simulink model "slrt_pmsm_2level_inverter"  (R2022b)
settings: Solver=FixedStepAuto  StartTime=0.0  StopTime=0.25  RelTol=1e-3  EnableMultiTasking=on
PreLoadFcn:
  | Ts = 1e-4;
  | Tcpu = 50e-6; %Controller sample time
  | 
  | % PMSM parameters
  | PM = 0.03; % Permanent magnet flux linkage
  | Ld = 2e-4;  % d-axis inductance
  | Lq = 2e-4;  % q-axis inductance
  | L0 = 2e-4;  % 0-axis inductance
  | Rs = 0.013; % Stator resistance
  | N = 6; % Number of pole pairs
  | J = 0.2; % Moment of inertia
  | 
  | % encoder parameters
  | numSlits = 2000; % number of slits
  | pulseSigOffset = 0; % index pulse signal offset
  | shaftInitPos = 0; % motor shaft initial position
  | 
  | % DAC parameters
  | gain = 0.1;
  | bias = 0;
  | 
  | % circuit parameters
  | Vdc = 48;
  | 
  | % real-time parameters
  | ts_FPGA_clk = 5e-9;
  | ts_FPGA_mdl = 1e-6;
  | 
  | % Real-time processor or embedded controller
  | RTorTTL = 1; % 1: Real-time processor,    0: embedded controller
  | 
  | % sample times
  | f_base = 200e6;
  | PWM_frequency = 20e3;
  | ts_FPGA_clk = 1/f_base;
  | ts_FPGA_mdl =1e-6;
libraries: simulink x5, hdlsllib x3, mcbhdlplantlib x2, slrtencoderlib x2, slrtresolverlib x2, slrthdlutillib x1, slrt2levelinverterlib x1
settings Model: Creator=chrisz  LastModifiedBy=chrisz
settings OptimizationCC: BlockReduction=off  ConditionallyExecuteInputs=off  DefaultParameterBehavior=Inlined
settings DebuggingCC: AlgebraicLoopMsg=error  SingleTaskRateTransMsg=error
settings HardwareCC: ProdBitPerPointer=32  ProdBitPerSizeT=32  ProdBitPerPtrDiffT=32  ProdLargestAtomicFloat=None  ProdIntDivRoundTo=Undefined  ProdEndianess=Unspecified  ProdWordSize=32  ProdHWDeviceType=ASIC/FPGA->ASIC/FPGA  TargetBitPerPointer=64  TargetBitPerSizeT=64  TargetBitPerPtrDiffT=64  TargetLongLongMode=on  TargetIntDivRoundTo=Zero  TargetEndianess=LittleEndian  TargetWordSize=64  TargetHWDeviceType=Custom Processor->MATLAB Host Computer  ProdEqTarget=off
settings ModelReferenceCC: EnableRefExpFcnMdlSchedulingChecks=on

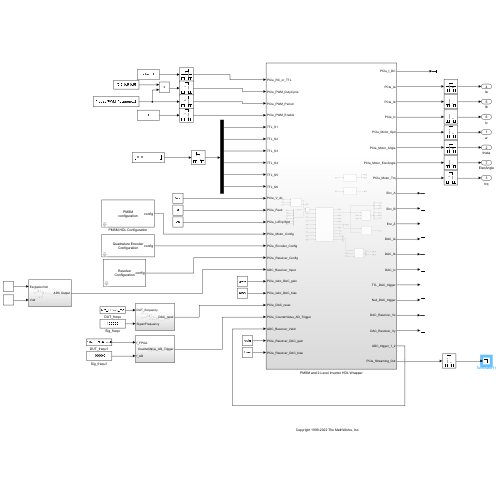
[thumbnail: Simulink's stored preview of the top-level diagram]
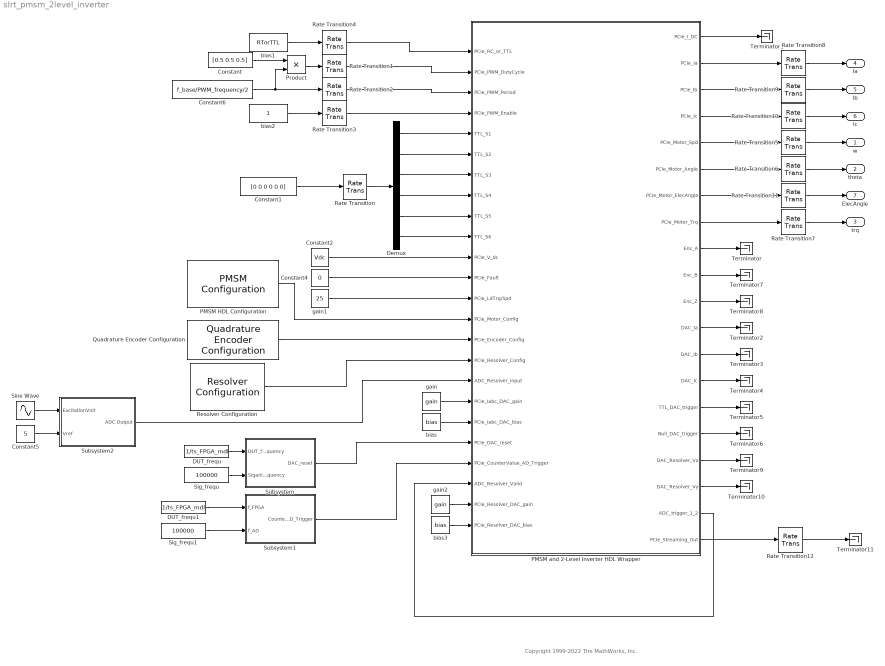
== system slrt_pmsm_2level_inverter ==
  note: Copyright 1999-2022 The MathWorks, Inc.
  Constant : Constant  Value=[0.5 0.5 0.5]  OutDataTypeStr=single  SampleTime=ts_FPGA_mdl
  Constant1 : Constant  Value=[0 0 0 0 0 0]  OutDataTypeStr=boolean  SampleTime=-1
  Constant2 : Constant  Value=Vdc  OutDataTypeStr=single  SampleTime=ts_FPGA_mdl
  Constant4 : Constant  Value=0  OutDataTypeStr=uint32  SampleTime=ts_FPGA_mdl
  Constant5 : Constant  Value=5  SampleTime=ts_FPGA_mdl
  Constant6 : Constant  Value=f_base/PWM_frequency/2  OutDataTypeStr=uint32  SampleTime=ts_FPGA_mdl
  DUT_frequ : Constant  Value=1/ts_FPGA_mdl  SampleTime=ts_FPGA_mdl
  DUT_frequ1 : Constant  Value=1/ts_FPGA_mdl  SampleTime=ts_FPGA_mdl
  Demux : Demux  Outputs=6
  PMSM HDL Configuration : mcbhdlplantlib/PMSM Configuration  portConfig=Torque  Trq_N_mode=0  Ts=1e-6  Pp=6  Rs=0.013  Ld=2e-4  Lq=2e-4  lambda_pm=0.03  J=0.2  B=4.924e-4  f=0
  PMSM and 2-Level Inverter HDL Wrapper : Subsystem
  Product : Product  OutDataTypeStr=uint32
  Quadrature Encoder Configuration : slrtencoderlib/Quadrature Encoder Configuration  NPulses=2000  zOffset=0  Ts=1e-6
  Rate Transition{,1..4} (5 alike) : RateTransition  OutPortSampleTime=ts_FPGA_clk
  Rate Transition{5..12} (8 alike) : RateTransition  OutPortSampleTime=Tcpu
  Resolver Configuration : slrtresolverlib/Resolver Configuration  Ts=1e-6  R=0.5  N=1  ADCrefV=5  ADCbits=16  totalADCCounts=65536
  Sig_frequ : Constant  Value=100000  VectorParams1D=off  SampleTime=ts_FPGA_mdl
  Sig_frequ1 : Constant  Value=100000  VectorParams1D=off  SampleTime=ts_FPGA_mdl
  Sine Wave : Sin  Amplitude=5  Frequency=62830  SampleTime=ts_FPGA_mdl
  Subsystem : Subsystem
  Subsystem1 : Subsystem
  Subsystem2 : Subsystem
  Terminator{,1..11} (12 alike) : Terminator
  bias : Constant  Value=bias  OutDataTypeStr=single  SampleTime=ts_FPGA_mdl
  bias1 : Constant  Value=RTorTTL  OutDataTypeStr=single  SampleTime=ts_FPGA_mdl
  bias2 : Constant  OutDataTypeStr=boolean  SampleTime=ts_FPGA_mdl
  bias3 : Constant  Value=bias  OutDataTypeStr=single  SampleTime=ts_FPGA_mdl
  gain : Constant  Value=gain  OutDataTypeStr=single  SampleTime=ts_FPGA_mdl
  gain1 : Constant  Value=25  OutDataTypeStr=single  SampleTime=ts_FPGA_mdl
  gain2 : Constant  Value=gain  OutDataTypeStr=single  SampleTime=ts_FPGA_mdl
  w : Outport
  theta : Outport  Port=2
  trq : Outport  Port=3
  Ia : Outport  Port=4
  Ib : Outport  Port=5
  Ic : Outport  Port=6
  ElecAngle : Outport  Port=7
  wires:
  bias1/1 -> Rate Transition4/1
  bias2/1 -> Rate Transition3/1
  Constant6/1 -> Product/2, Rate Transition2/1
  Product/1 -> Rate Transition1/1
  Constant/1 -> Product/1
  gain/1 -> PMSM and 2-Level Inverter HDL Wrapper/18(PCIe_Iabc_DAC_gain)
  bias/1 -> PMSM and 2-Level Inverter HDL Wrapper/19(PCIe_Iabc_DAC_bias)
  Rate Transition4/1 -> PMSM and 2-Level Inverter HDL Wrapper/1(PCIe_RC_or_TTL)
  Rate Transition3/1 -> PMSM and 2-Level Inverter HDL Wrapper/4(PCIe_PWM_Enable)
  Rate Transition2/1 -> PMSM and 2-Level Inverter HDL Wrapper/3(PCIe_PWM_Period)
  Rate Transition1/1 -> PMSM and 2-Level Inverter HDL Wrapper/2(PCIe_PWM_DutyCycle)
  Rate Transition/1 -> Demux/1
  Demux/1 -> PMSM and 2-Level Inverter HDL Wrapper/5(TTL_S1)
  Demux/2 -> PMSM and 2-Level Inverter HDL Wrapper/6(TTL_S2)
  Demux/3 -> PMSM and 2-Level Inverter HDL Wrapper/7(TTL_S3)
  Demux/4 -> PMSM and 2-Level Inverter HDL Wrapper/8(TTL_S4)
  Demux/5 -> PMSM and 2-Level Inverter HDL Wrapper/9(TTL_S5)
  Demux/6 -> PMSM and 2-Level Inverter HDL Wrapper/10(TTL_S6)
  Constant1/1 -> Rate Transition/1
  Constant2/1 -> PMSM and 2-Level Inverter HDL Wrapper/11(PCIe_V_dc)
  Constant4/1 -> PMSM and 2-Level Inverter HDL Wrapper/12(PCIe_Fault)
  gain1/1 -> PMSM and 2-Level Inverter HDL Wrapper/13(PCIe_LdTrq/Spd)
  DUT_frequ/1 -> Subsystem/1(DUT_frequency)
  Sig_frequ/1 -> Subsystem/2(SiganlFrequency)
  Subsystem/1(DAC_reset) -> PMSM and 2-Level Inverter HDL Wrapper/20(PCIe_DAC_reset)
  Rate Transition6/1 -> theta/1
  PMSM and 2-Level Inverter HDL Wrapper/9(Enc_A) -> Terminator/1
  Rate Transition7/1 -> trq/1
  PMSM and 2-Level Inverter HDL Wrapper/12(DAC_Ia) -> Terminator2/1
  PMSM and 2-Level Inverter HDL Wrapper/1(PCIe_I_DC) -> Terminator1/1
  PMSM and 2-Level Inverter HDL Wrapper/10(Enc_B) -> Terminator7/1
  PMSM and 2-Level Inverter HDL Wrapper/14(DAC_Ic) -> Terminator4/1
  Rate Transition5/1 -> w/1
  Rate Transition10/1 -> Ic/1
  PMSM and 2-Level Inverter HDL Wrapper/15(TTL_DAC_trigger) -> Terminator5/1
  PMSM and 2-Level Inverter HDL Wrapper/13(DAC_Ib) -> Terminator3/1
  PMSM and 2-Level Inverter HDL Wrapper/16(Null_DAC_trigger) -> Terminator6/1
  Rate Transition9/1 -> Ib/1
  Rate Transition8/1 -> Ia/1
  PMSM and 2-Level Inverter HDL Wrapper/5(PCIe_Motor_Spd) -> Rate Transition5/1
  PMSM and 2-Level Inverter HDL Wrapper/6(PCIe_Motor_Angle) -> Rate Transition6/1
  PMSM and 2-Level Inverter HDL Wrapper/8(PCIe_Motor_Trq) -> Rate Transition7/1
  PMSM and 2-Level Inverter HDL Wrapper/2(PCIe_Ia) -> Rate Transition8/1
  PMSM and 2-Level Inverter HDL Wrapper/3(PCIe_Ib) -> Rate Transition9/1
  PMSM and 2-Level Inverter HDL Wrapper/4(PCIe_Ic) -> Rate Transition10/1
  PMSM and 2-Level Inverter HDL Wrapper/11(Enc_Z) -> Terminator8/1
  PMSM and 2-Level Inverter HDL Wrapper/17(DAC_Resolver_Vx) -> Terminator9/1
  PMSM and 2-Level Inverter HDL Wrapper/18(DAC_Resolver_Vy) -> Terminator10/1
  Quadrature Encoder Configuration/1 -> PMSM and 2-Level Inverter HDL Wrapper/15(PCIe_Encoder_Config)
  PMSM HDL Configuration/1 -> PMSM and 2-Level Inverter HDL Wrapper/14(PCIe_Motor_Config)
  Resolver Configuration/1 -> PMSM and 2-Level Inverter HDL Wrapper/16(PCIe_Resolver_Config)
  Subsystem1/1(CounterValue_AD_Trigger) -> PMSM and 2-Level Inverter HDL Wrapper/21(PCIe_CounterValue_AD_Trigger)
  PMSM and 2-Level Inverter HDL Wrapper/19(ADC_trigger_1_2) -> PMSM and 2-Level Inverter HDL Wrapper/22(ADC_Resolver_Valid)
  Sig_frequ1/1 -> Subsystem1/2(f_AD)
  DUT_frequ1/1 -> Subsystem1/1(f_FPGA)
  Sine Wave/1 -> Subsystem2/1(ExcitationVolt)
  Constant5/1 -> Subsystem2/2(Vref)
  Subsystem2/1(ADC Output) -> PMSM and 2-Level Inverter HDL Wrapper/17(ADC_Resolver_Input)
  Rate Transition11/1 -> ElecAngle/1
  PMSM and 2-Level Inverter HDL Wrapper/7(PCIe_Motor_ElecAngle) -> Rate Transition11/1
  gain2/1 -> PMSM and 2-Level Inverter HDL Wrapper/23(PCIe_Resolver_DAC_gain)
  bias3/1 -> PMSM and 2-Level Inverter HDL Wrapper/24(PCIe_Resolver_DAC_bias)
  PMSM and 2-Level Inverter HDL Wrapper/20(PCIe_Streaming_Out) -> Rate Transition12/1
  Rate Transition12/1 -> Terminator11/1

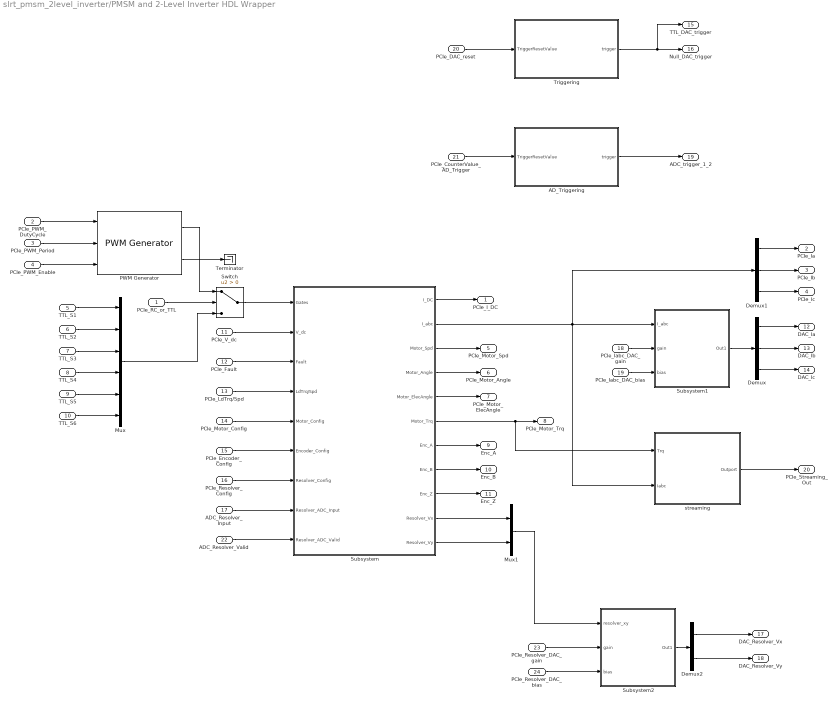
== system slrt_pmsm_2level_inverter/PMSM and 2-Level Inverter HDL Wrapper ==
  PCIe_RC_or_TTL : Inport
  PCIe_PWM_DutyCycle : Inport  Port=2
  PCIe_PWM_Period : Inport  Port=3
  PCIe_PWM_Enable : Inport  Port=4
  TTL_S1 : Inport  Port=5
  TTL_S2 : Inport  Port=6
  TTL_S3 : Inport  Port=7
  TTL_S4 : Inport  Port=8
  TTL_S5 : Inport  Port=9
  TTL_S6 : Inport  Port=10
  PCIe_V_dc : Inport  Port=11
  PCIe_Fault : Inport  Port=12
  PCIe_LdTrq/Spd : Inport  Port=13
  PCIe_Motor_Config : Inport  Port=14
  PCIe_Encoder_Config : Inport  Port=15
  PCIe_Resolver_Config : Inport  Port=16
  ADC_Resolver_Input : Inport  Port=17
  PCIe_Iabc_DAC_gain : Inport  Port=18
  PCIe_Iabc_DAC_bias : Inport  Port=19
  PCIe_DAC_reset : Inport  Port=20
  PCIe_CounterValue_AD_Trigger : Inport  Port=21  OutDataTypeStr=uint32
  ADC_Resolver_Valid : Inport  Port=22
  PCIe_Resolver_DAC_gain : Inport  Port=23
  PCIe_Resolver_DAC_bias : Inport  Port=24
  AD_Triggering : Subsystem
  Demux : Demux  Outputs=3
  Demux1 : Demux  Outputs=3
  Demux2 : Demux  Outputs=2
  Mux : Mux  Inputs=6
  Mux1 : Mux  Inputs=2
  PWM Generator : slrthdlutillib/PWM Generator
  Subsystem : Subsystem
  Subsystem1 : Subsystem
  Subsystem2 : Subsystem
  Switch : Switch  Criteria=u2 > Threshold  SaturateOnIntegerOverflow=off  InputSameDT=off
  Terminator : Terminator
  Triggering : Subsystem
  streaming : Subsystem
  PCIe_I_DC : Outport
  PCIe_Ia : Outport  Port=2
  PCIe_Ib : Outport  Port=3
  PCIe_Ic : Outport  Port=4
  PCIe_Motor_Spd : Outport  Port=5
  PCIe_Motor_Angle : Outport  Port=6
  PCIe_Motor_ElecAngle : Outport  Port=7
  PCIe_Motor_Trq : Outport  Port=8
  Enc_A : Outport  Port=9
  Enc_B : Outport  Port=10
  Enc_Z : Outport  Port=11
  DAC_Ia : Outport  Port=12
  DAC_Ib : Outport  Port=13
  DAC_Ic : Outport  Port=14
  TTL_DAC_trigger : Outport  Port=15
  Null_DAC_trigger : Outport  Port=16
  DAC_Resolver_Vx : Outport  Port=17
  DAC_Resolver_Vy : Outport  Port=18
  ADC_trigger_1_2 : Outport  Port=19  OutDataTypeStr=boolean
  PCIe_Streaming_Out : Outport  Port=20
  wires:
  Subsystem/7(Enc_A) -> Enc_A/1
  TTL_S2/1 -> Mux/2
  Demux1/1 -> PCIe_Ia/1
  PCIe_PWM_DutyCycle/1 -> PWM Generator/1
  TTL_S5/1 -> Mux/5
  Subsystem/2(I_abc) -> Demux1/1, streaming/2(Iabc), Subsystem1/1(I_abc)
  Subsystem/6(Motor_Trq) -> streaming/1(Trq), PCIe_Motor_Trq/1
  Subsystem/4(Motor_Angle) -> PCIe_Motor_Angle/1
  Subsystem/1(I_DC) -> PCIe_I_DC/1
  PCIe_Encoder_Config/1 -> Subsystem/6(Encoder_Config)
  PCIe_Iabc_DAC_bias/1 -> Subsystem1/3(bias)
  Subsystem/3(Motor_Spd) -> PCIe_Motor_Spd/1
  Subsystem/8(Enc_B) -> Enc_B/1
  PCIe_V_dc/1 -> Subsystem/2(V_dc)
  PWM Generator/1 -> Switch/1
  Triggering/1(trigger) -> Null_DAC_trigger/1, TTL_DAC_trigger/1
  TTL_S6/1 -> Mux/6
  Subsystem/9(Enc_Z) -> Enc_Z/1
  PCIe_LdTrq/Spd/1 -> Subsystem/4(LdTrq/Spd)
  TTL_S1/1 -> Mux/1
  Demux1/3 -> PCIe_Ic/1
  Demux1/2 -> PCIe_Ib/1
  PCIe_RC_or_TTL/1 -> Switch/2
  PCIe_Motor_Config/1 -> Subsystem/5(Motor_Config)
  Demux/1 -> DAC_Ia/1
  Mux/1 -> Switch/3
  PCIe_PWM_Period/1 -> PWM Generator/2
  TTL_S4/1 -> Mux/4
  PCIe_Fault/1 -> Subsystem/3(Fault)
  PCIe_DAC_reset/1 -> Triggering/1(TriggerResetValue)
  PCIe_Iabc_DAC_gain/1 -> Subsystem1/2(gain)
  PCIe_PWM_Enable/1 -> PWM Generator/3
  Demux/2 -> DAC_Ib/1
  Switch/1 -> Subsystem/1(Gates)
  Subsystem1/1(Out1) -> Demux/1
  TTL_S3/1 -> Mux/3
  Demux/3 -> DAC_Ic/1
  PCIe_Resolver_Config/1 -> Subsystem/7(Resolver_Config)
  ADC_Resolver_Input/1 -> Subsystem/8(Resolver_ADC_Input)
  PCIe_CounterValue_AD_Trigger/1 -> AD_Triggering/1(TriggerResetValue)
  AD_Triggering/1(trigger) -> ADC_trigger_1_2/1
  ADC_Resolver_Valid/1 -> Subsystem/9(Resolver_ADC_Valid)
  Subsystem/5(Motor_ElecAngle) -> PCIe_Motor_ElecAngle/1
  streaming/1(Outport) -> PCIe_Streaming_Out/1
  Subsystem/10(Resolver_Vx) -> Mux1/1
  Subsystem/11(Resolver_Vy) -> Mux1/2
  Mux1/1 -> Subsystem2/1(resolver_xy)
  PCIe_Resolver_DAC_gain/1 -> Subsystem2/2(gain)
  PCIe_Resolver_DAC_bias/1 -> Subsystem2/3(bias)
  Subsystem2/1(Out1) -> Demux2/1
  Demux2/1 -> DAC_Resolver_Vx/1
  Demux2/2 -> DAC_Resolver_Vy/1
  PWM Generator/2 -> Terminator/1

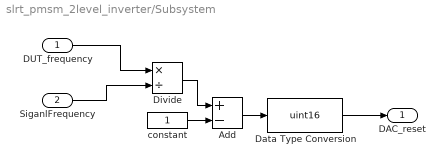
== system slrt_pmsm_2level_inverter/Subsystem ==
  DUT_frequency : Inport
  SiganlFrequency : Inport  Port=2
  Add : Sum  Inputs=+-
  Data Type Conversion : DataTypeConversion  OutDataTypeStr=uint16  SaturateOnIntegerOverflow=off  RndMeth=Floor
  Divide : Product  Inputs=*/
  constant : Constant  VectorParams1D=off  SampleTime=-1
  DAC_reset : Outport
  wires:
  DUT_frequency/1 -> Divide/1
  constant/1 -> Add/2
  Data Type Conversion/1 -> DAC_reset/1
  Divide/1 -> Add/1
  Add/1 -> Data Type Conversion/1
  SiganlFrequency/1 -> Divide/2

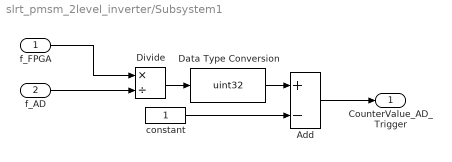
== system slrt_pmsm_2level_inverter/Subsystem1 ==
  f_FPGA : Inport
  f_AD : Inport  Port=2
  Add : Sum  Inputs=+-  AccumDataTypeStr=uint32
  Data Type Conversion : DataTypeConversion  OutDataTypeStr=uint32  SaturateOnIntegerOverflow=off  RndMeth=Floor
  Divide : Product  Inputs=*/
  constant : Constant  VectorParams1D=off  OutDataTypeStr=uint32  SampleTime=-1
  CounterValue_AD_Trigger : Outport
  wires:
  f_AD/1 -> Divide/2
  f_FPGA/1 -> Divide/1
  Divide/1 -> Data Type Conversion/1
  Data Type Conversion/1 -> Add/1
  constant/1 -> Add/2
  Add/1 -> CounterValue_AD_Trigger/1

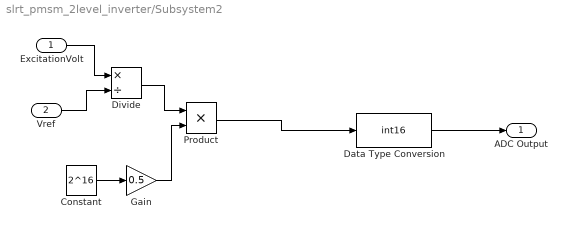
== system slrt_pmsm_2level_inverter/Subsystem2 ==
  ExcitationVolt : Inport
  Vref : Inport  Port=2
  Constant : Constant  Value=2^16  SampleTime=-1
  Data Type Conversion : DataTypeConversion  OutDataTypeStr=int16  RndMeth=Nearest
  Divide : Product  Inputs=*/
  Gain : Gain  Gain=0.5
  Product : Product
  ADC Output : Outport
  wires:
  ExcitationVolt/1 -> Divide/1
  Vref/1 -> Divide/2
  Constant/1 -> Gain/1
  Divide/1 -> Product/1
  Gain/1 -> Product/2
  Product/1 -> Data Type Conversion/1
  Data Type Conversion/1 -> ADC Output/1

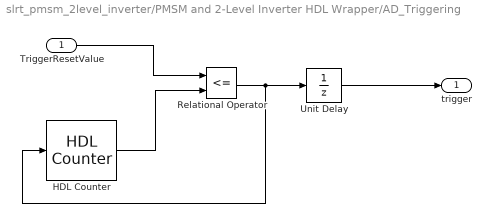
== system slrt_pmsm_2level_inverter/PMSM and 2-Level Inverter HDL Wrapper/AD_Triggering ==
  TriggerResetValue : Inport
  HDL Counter : hdlsllib/Sources/HDL Counter  CountType=Free running  CountInit=0  CountStep=1  CountMax=25  CountFromType=Initial value  CountFrom=0  CountResetPort=on  CountLoadPort=off  CountEnbPort=off  CountDirPort=off  CountHitOutputPort=off  CountDataType=Unsigned  CountWordLen=32  CountFracLen=0  CountSampTime=1
  Relational Operator : RelationalOperator  Operator=<=  OutDataTypeStr=boolean  InputSameDT=off
  Unit Delay : UnitDelay  SampleTime=-1  HasFrameUpgradeWarning=on
  trigger : Outport
  wires:
  TriggerResetValue/1 -> Relational Operator/1
  HDL Counter/1 -> Relational Operator/2
  Relational Operator/1 -> HDL Counter/1, Unit Delay/1
  Unit Delay/1 -> trigger/1

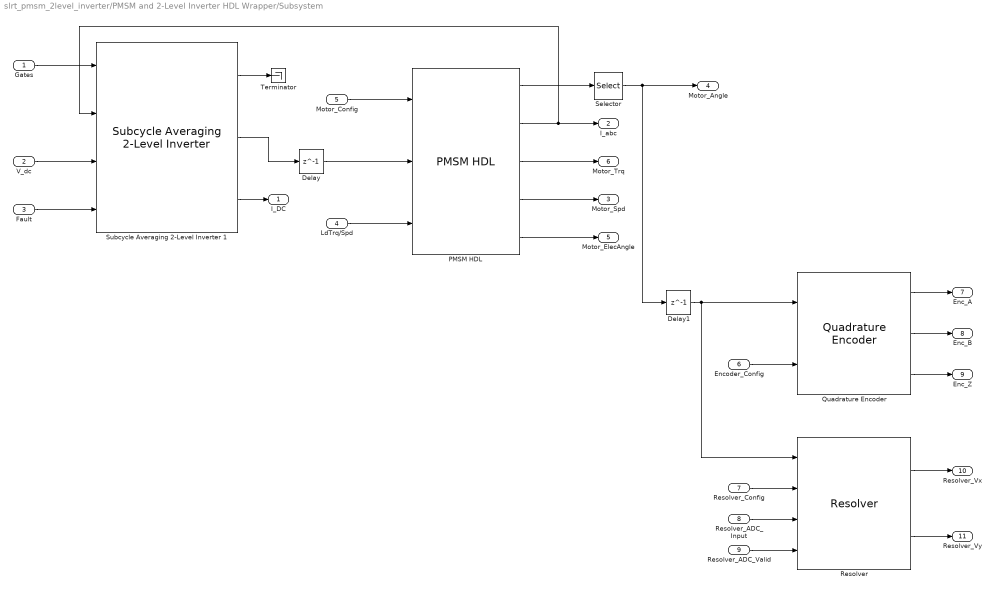
== system slrt_pmsm_2level_inverter/PMSM and 2-Level Inverter HDL Wrapper/Subsystem ==
  Gates : Inport
  V_dc : Inport  Port=2
  Fault : Inport  Port=3
  LdTrq/Spd : Inport  Port=4
  Motor_Config : Inport  Port=5
  Encoder_Config : Inport  Port=6
  Resolver_Config : Inport  Port=7
  Resolver_ADC_Input : Inport  Port=8
  Resolver_ADC_Valid : Inport  Port=9
  Delay : Delay  DelayLength=1
  Delay1 : Delay  DelayLength=1
  PMSM HDL : mcbhdlplantlib/PMSM HDL  VariantControl=pmsmVariant==pmsmEnum.TorqueInput  Ts=1e-6
  Quadrature Encoder : slrtencoderlib/Quadrature Encoder
  Resolver : slrtresolverlib/Resolver  Ts=ts_FPGA_mdl
  Selector : Selector  InputPortWidth=14  IndexOptions=Index vector (dialog)  Indices=[10]  OutputSizes=1
  Subcycle Averaging 2-Level Inverter 1 : slrt2levelinverterlib/Subcycle Averaging 2-Level Inverter   rSwitch=0.001  vfSwitch=0.1  rDiode=0.001  vfDiode=0.8  rSnub=100  ts_Model=ts_FPGA_mdl  ts_FPGA=ts_FPGA_clk
  Terminator : Terminator
  I_DC : Outport
  I_abc : Outport  Port=2
  Motor_Spd : Outport  Port=3
  Motor_Angle : Outport  Port=4
  Motor_ElecAngle : Outport  Port=5
  Motor_Trq : Outport  Port=6
  Enc_A : Outport  Port=7
  Enc_B : Outport  Port=8
  Enc_Z : Outport  Port=9
  Resolver_Vx : Outport  Port=10
  Resolver_Vy : Outport  Port=11
  wires:
  Motor_Config/1 -> PMSM HDL/1
  Subcycle Averaging 2-Level Inverter 1/3 -> I_DC/1
  V_dc/1 -> Subcycle Averaging 2-Level Inverter 1/3
  PMSM HDL/2 -> Subcycle Averaging 2-Level Inverter 1/2, I_abc/1
  Quadrature Encoder/2 -> Enc_B/1
  Fault/1 -> Subcycle Averaging 2-Level Inverter 1/4
  Quadrature Encoder/1 -> Enc_A/1
  PMSM HDL/3 -> Motor_Trq/1
  LdTrq/Spd/1 -> PMSM HDL/3
  Quadrature Encoder/3 -> Enc_Z/1
  PMSM HDL/4 -> Motor_Spd/1
  Encoder_Config/1 -> Quadrature Encoder/2
  Gates/1 -> Subcycle Averaging 2-Level Inverter 1/1
  Resolver_Config/1 -> Resolver/2
  Resolver_ADC_Input/1 -> Resolver/3
  Resolver/1 -> Resolver_Vx/1
  Resolver/2 -> Resolver_Vy/1
  Resolver_ADC_Valid/1 -> Resolver/4
  Subcycle Averaging 2-Level Inverter 1/1 -> Terminator/1
  PMSM HDL/1 -> Selector/1
  PMSM HDL/5 -> Motor_ElecAngle/1
  Subcycle Averaging 2-Level Inverter 1/2 -> Delay/1
  Delay/1 -> PMSM HDL/2
  Selector/1 -> Delay1/1, Motor_Angle/1
  Delay1/1 -> Resolver/1, Quadrature Encoder/1

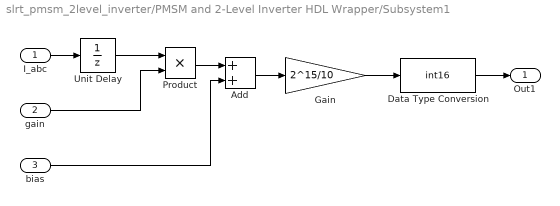
== system slrt_pmsm_2level_inverter/PMSM and 2-Level Inverter HDL Wrapper/Subsystem1 ==
  I_abc : Inport
  gain : Inport  Port=2
  bias : Inport  Port=3
  Add : Sum
  Data Type Conversion : DataTypeConversion  OutDataTypeStr=int16  SaturateOnIntegerOverflow=off  RndMeth=Floor
  Gain : Gain  Gain=2^15/10
  Product : Product
  Unit Delay : UnitDelay  SampleTime=-1  HasFrameUpgradeWarning=on
  Out1 : Outport
  wires:
  I_abc/1 -> Unit Delay/1
  Unit Delay/1 -> Product/1
  gain/1 -> Product/2
  Product/1 -> Add/1
  bias/1 -> Add/2
  Add/1 -> Gain/1
  Gain/1 -> Data Type Conversion/1
  Data Type Conversion/1 -> Out1/1

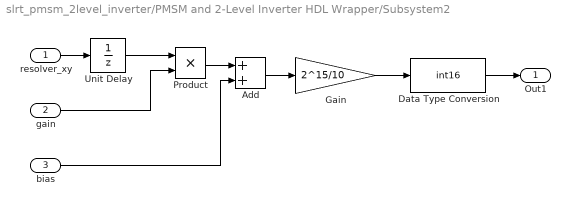
== system slrt_pmsm_2level_inverter/PMSM and 2-Level Inverter HDL Wrapper/Subsystem2 ==
  resolver_xy : Inport
  gain : Inport  Port=2
  bias : Inport  Port=3
  Add : Sum
  Data Type Conversion : DataTypeConversion  OutDataTypeStr=int16  SaturateOnIntegerOverflow=off  RndMeth=Floor
  Gain : Gain  Gain=2^15/10
  Product : Product
  Unit Delay : UnitDelay  SampleTime=-1  HasFrameUpgradeWarning=on
  Out1 : Outport
  wires:
  resolver_xy/1 -> Unit Delay/1
  Unit Delay/1 -> Product/1
  gain/1 -> Product/2
  Product/1 -> Add/1
  bias/1 -> Add/2
  Add/1 -> Gain/1
  Gain/1 -> Data Type Conversion/1
  Data Type Conversion/1 -> Out1/1

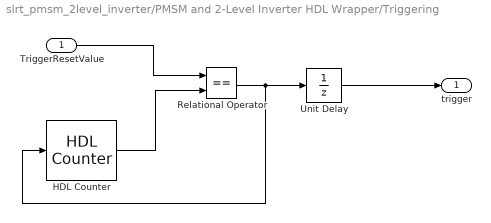
== system slrt_pmsm_2level_inverter/PMSM and 2-Level Inverter HDL Wrapper/Triggering ==
  TriggerResetValue : Inport
  HDL Counter : hdlsllib/Sources/HDL Counter  CountType=Free running  CountInit=0  CountStep=1  CountMax=25  CountFromType=Initial value  CountFrom=0  CountResetPort=on  CountLoadPort=off  CountEnbPort=off  CountDirPort=off  CountHitOutputPort=off  CountDataType=Unsigned  CountWordLen=16  CountFracLen=0  CountSampTime=1
  Relational Operator : RelationalOperator  Operator===  OutDataTypeStr=boolean  InputSameDT=off
  Unit Delay : UnitDelay  SampleTime=-1  HasFrameUpgradeWarning=on
  trigger : Outport
  wires:
  TriggerResetValue/1 -> Relational Operator/1
  HDL Counter/1 -> Relational Operator/2
  Relational Operator/1 -> HDL Counter/1, Unit Delay/1
  Unit Delay/1 -> trigger/1

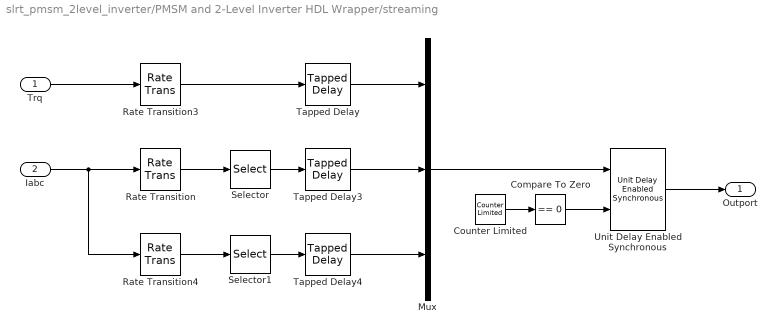
== system slrt_pmsm_2level_inverter/PMSM and 2-Level Inverter HDL Wrapper/streaming ==
  Trq : Inport
  Iabc : Inport  Port=2
  Compare To Zero : simulink/Logic and Bit Operations/Compare To Zero  relop===  OutDataTypeStr=boolean
  Counter Limited : simulink/Sources/Counter Limited  uplimit=49  tsamp=ts_FPGA_mdl
  Mux : Mux  Inputs=3
  Rate Transition : RateTransition
  Rate Transition3 : RateTransition
  Rate Transition4 : RateTransition
  Selector : Selector  InputPortWidth=3  IndexOptions=Index vector (dialog)  Indices=[1]  OutputSizes=1
  Selector1 : Selector  InputPortWidth=3  IndexOptions=Index vector (dialog)  Indices=[2]  OutputSizes=1
  Tapped Delay : simulink/Discrete/Tapped Delay  vinit=0.0  samptime=ts_FPGA_mdl  NumDelays=50  DelayOrder=Oldest  includeCurrent=off
  Tapped Delay3 : simulink/Discrete/Tapped Delay  vinit=0.0  samptime=ts_FPGA_mdl  NumDelays=50  DelayOrder=Oldest  includeCurrent=off
  Tapped Delay4 : simulink/Discrete/Tapped Delay  vinit=0.0  samptime=ts_FPGA_mdl  NumDelays=50  DelayOrder=Oldest  includeCurrent=off
  Unit Delay Enabled Synchronous : hdlsllib/Discrete/Unit Delay Enabled Synchronous  InitialCondition=0.0  SampleTime=-1
  Outport : Outport
  wires:
  Iabc/1 -> Rate Transition4/1, Rate Transition/1
  Trq/1 -> Rate Transition3/1
  Rate Transition3/1 -> Tapped Delay/1
  Rate Transition/1 -> Selector/1
  Rate Transition4/1 -> Selector1/1
  Selector/1 -> Tapped Delay3/1
  Selector1/1 -> Tapped Delay4/1
  Tapped Delay/1 -> Mux/1
  Tapped Delay3/1 -> Mux/2
  Tapped Delay4/1 -> Mux/3
  Mux/1 -> Unit Delay Enabled Synchronous/1
  Counter Limited/1 -> Compare To Zero/1
  Compare To Zero/1 -> Unit Delay Enabled Synchronous/2
  Unit Delay Enabled Synchronous/1 -> Outport/1
